simulink subsystem "Actuator"  (R2023a)
settings: Solver=VariableStepAuto  StartTime=0.0  StopTime=10.0  RelTol=1e-3
model mask{K=12, Kv=2, K1=0, K2=0, K3=0}
  mask prompts: K "Main gain cofficient"; Kv "Velocity gain cofficient"; K1 "Acceleration gain cofficient"; K2 "Some parameter"; K3 "Some another parameter"
settings Model: Creator=maxim  LastModifiedBy=Artem Sannikov

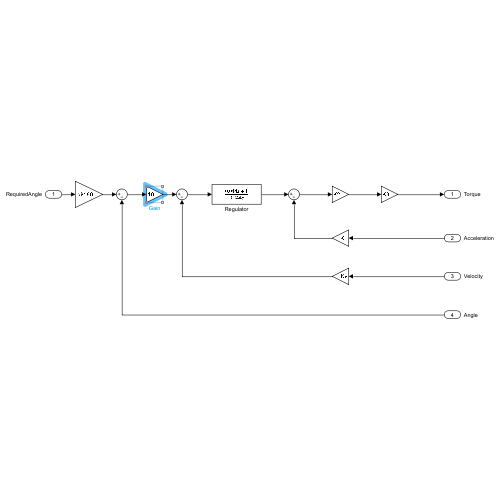
[thumbnail: Simulink's stored preview of the top-level diagram]
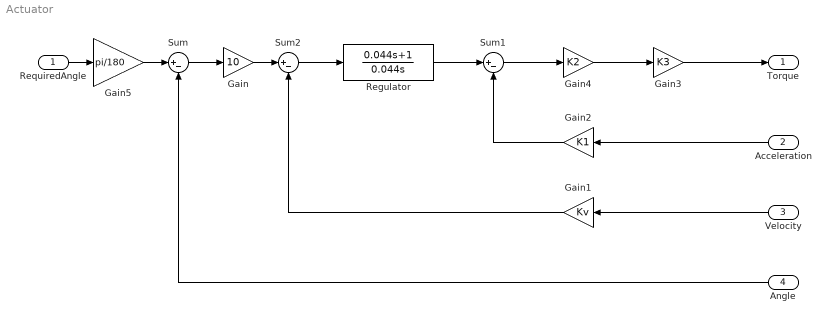
== system Actuator ==
  RequiredAngle : Inport
  Acceleration : Inport  Port=2
  Velocity : Inport  Port=3
  Angle : Inport  Port=4
  Gain : Gain  Gain=10
  Gain1 : Gain  Gain=Kv
  Gain2 : Gain  Gain=K1
  Gain3 : Gain  Gain=K3
  Gain4 : Gain  Gain=K2
  Gain5 : Gain  Gain=pi/180
  Regulator : TransferFcn  Numerator=[0.044 1]  Denominator=[0.044 0]
  Sum : Sum  Inputs=|+-
  Sum1 : Sum  Inputs=|+-
  Sum2 : Sum  Inputs=|+-
  Torque : Outport
  wires:
  RequiredAngle/1 -> Gain5/1
  Sum/1 -> Gain/1
  Gain/1 -> Sum2/1
  Regulator/1 -> Sum1/1
  Sum1/1 -> Gain4/1
  Gain4/1 -> Gain3/1
  Gain2/1 -> Sum1/2
  Gain1/1 -> Sum2/2
  Gain3/1 -> Torque/1
  Acceleration/1 -> Gain2/1
  Velocity/1 -> Gain1/1
  Sum2/1 -> Regulator/1
  Angle/1 -> Sum/2
  Gain5/1 -> Sum/1
